simulink model "omegaController"  (R2019a)
settings: Solver=VariableStepAuto  StartTime=0.0  StopTime=10.0  RelTol=1e-3
values from neighbouring files (symbols this model uses):
  alpha0 = 0.01    [forces_moments.m]    (also in forces_moments_testing.m; omegaController.m; precisionLanding.m)
  Maabb = [P.C_ell_beta 0; 0 P.C_m_alpha; P.C_n_beta 0]    [forces_moments.m]    (also in forces_moments_testing.m; omegaController.m; precisionLanding.m)
  Mdd = [0,P.C_ell_delta_a,P.C_ell_delta_r ... (first row only)    [forces_moments.m]    (also in forces_moments_testing.m; omegaController.m; precisionLanding.m)
  Moo = Moo/(2*V)    [forces_moments.m]    (also in forces_moments_testing.m; omegaController.m; precisionLanding.m)
settings Model: Creator=josea  LastModifiedBy=pedro
settings DataIOCC: ReturnWorkspaceOutputs=off
settings DebuggingCC: PregeneratedLibrarySubsystemCodeDiagnostic=none  ArithmeticOperatorsInVariantConditions=warning
settings SFSimCC: SimUseLocalCustomCode=off
settings RTWCC: RTWUseLocalCustomCode=off

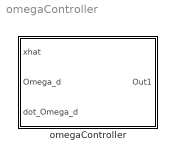
== system omegaController ==
  omegaController : Subsystem

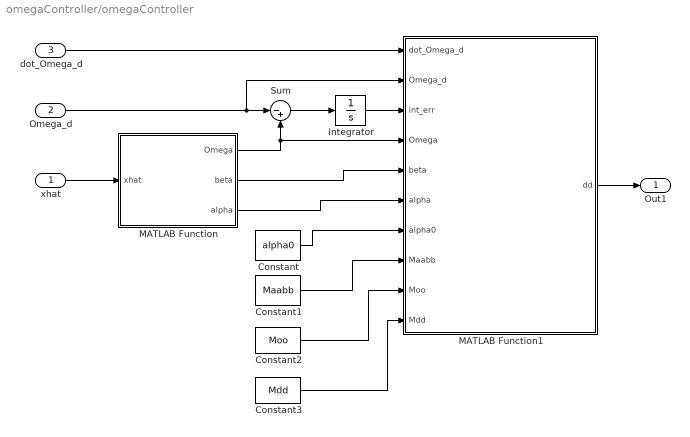
== system omegaController/omegaController ==
  xhat : Inport
  Omega_d : Inport  Port=2
  dot_Omega_d : Inport  Port=3
  Constant : Constant  Value=alpha0
  Constant1 : Constant  Value=Maabb
  Constant2 : Constant  Value=Moo
  Constant3 : Constant  Value=Mdd
  Integrator : Integrator
  MATLAB Function : MATLAB Function  TreatAsAtomicUnit=on
  MATLAB Function1 : MATLAB Function  TreatAsAtomicUnit=on
  Sum : Sum  Inputs=|-+
  Out1 : Outport
  wires:
  xhat/1 -> MATLAB Function/1(xhat)
  Omega_d/1 -> MATLAB Function1/2(Omega_d), Sum/1
  Sum/1 -> Integrator/1
  MATLAB Function/1(Omega) -> Sum/2, MATLAB Function1/4(Omega)
  MATLAB Function/3(alpha) -> MATLAB Function1/6(alpha)
  MATLAB Function/2(beta) -> MATLAB Function1/5(beta)
  Integrator/1 -> MATLAB Function1/3(int_err)
  dot_Omega_d/1 -> MATLAB Function1/1(dot_Omega_d)
  MATLAB Function1/1(dd) -> Out1/1
  Constant/1 -> MATLAB Function1/7(alpha0)
  Constant1/1 -> MATLAB Function1/8(Maabb)
  Constant2/1 -> MATLAB Function1/9(Moo)
  Constant3/1 -> MATLAB Function1/10(Mdd)

== matlab function omegaController/MATLAB Function1 ==
  data: dot_Omega_d input; Omega_d input; int_err input; Omega input; beta input; alpha input; alpha0 input; Maabb input; dd output; Moo input; Mdd input
function dd = controller(dot_Omega_d,Omega_d,int_err,Omega,beta,alpha,alpha0,Maabb,Moo,Mdd)
% Equation 48 [1]

    % gains
    kp = 1;
    ki = 1;
    
    % auxiliary calculations
    Soo = skew(Omega);
    
    % control law
    dd = Mdd\(Soo*Omega-...
        Maabb*[beta;alpha-alpha0]-...
        Moo*Omega-...
        kp*(Omega-Omega_d)-...
        ki*int_err+dot_Omega_d);
end

function S = skew(vector)
    S = [0,-vector(3),vector(2);
        vector(3),0,-vector(1);
        -vector(2),vector(1),0];
end

% [1] Serra, Pedro & Cunha, Rita & Hamel, T. & Silvestre, Carlos & Le Bras, Florent. (2015). Nonlinear Image-Based Visual Servo Controller for the Flare Maneuver of Fixed-Wing Aircraft Using Optical Flow. IEEE Transactions on Control Systems Technology. 23. 570–583. 10.1109/TCST.2014.2330996.

== matlab function omegaController/MATLAB Function ==
  data: xhat input; Omega output; beta output; alpha output
function [Omega,beta,alpha] = getData(xhat)
    Omega = xhat(10:12);
    beta = xhat(6);
    alpha = xhat(5);
end
